simulink model "crf_ut"  (Simulink 8.1)
settings: Solver=FixedStepDiscrete  StartTime=0.0  StopTime=10  FixedStep=0.005  RelTol=1e-3
PostLoadFcn:
  | , if any(exist('dsrtsu_mdlpostloadfcn', 'file') == [2, 3, 6]), try dsrtsu_mdlpostloadfcn('Execute', bdroot); catch fprintf('Error in PostLoadFcn (dsrtsu_mdlpostloadfcn) for model "%s":\n %s\n', bdroot, lasterr); end, end,
libraries: siltestlib x9, crf x1
settings Model: DSRTSU_INTERNAL_RTI_VER=450  DSRTSU_INTERNAL_RTI_TYPE=rti1401  RTICANMMDATA=struct('GeneralSetupData',struct('modelroot','D:\ELN150201_TAIWAN\trunk\AdasDragon\software\sw_development\arch\app\jud','generalsettings',struct('filesettings',struct('destfolder',struct('Name','RTICANMM_FILES','Check',1),'buildfolder',struct('Name','.','Check',1),'AbsDestfolder',struct('Name','D:\ELN150201_TAIWAN\trunk\AdasDragon\software\sw_development\arch\app\jud\RTICANMM_FILES'),'AbsBuildfolder',struct('Name','D:\ELN150201_TAIWAN\trunk\AdasDragon\software\sw_development\arch\app\jud'))),'options',struct('addpaths',1,'rmpaths',1,'addtrcexclusion',logical(1),'cannavigator',struct('checkmonitoring',0),'show_usrtrc',0,'use_usrtrc',0),'advanced',struct('options',[1 1 1 1 1 1 1 1 1 1 1 1 1 1 1 1 1 1 1 1 1 1 1 1 1 1 1 1 1 1 1 1 1 1 1 1 1 1 1 1 1 1 1 1 1 1 1 1 1 1 1 1 1 1 1 1 1 1 1 1 1 1 1 1 1 1 1 1 1 1 1 1 1 1 1 1 1 1 1 1 1 1 1 1 1 1 1 1 1 1 1 1 1 1 1 1 1 1 1 1]),'MPSetup',{{}},'modelname','crf_ut','block','crf_ut'))  DSRTSU_INTERNAL_RTIFPGA=40  Creator=AT015411  LastModifiedBy=AT015555  BufferReuse=off
settings DataIOCC: SignalLoggingSaveFormat=Dataset
settings OptimizationCC: BlockReduction=off  OptimizeBlockIOStorage=off  BufferReuse=off  ExpressionFolding=off  ExpressionDepthLimit=128  LocalBlockOutputs=off
settings DebuggingCC: FcnCallInpInsideContextMsg=EnableAllAsError
settings HardwareCC: ProdIntDivRoundTo=Zero  ProdEndianess=BigEndian  ProdHWDeviceType=Generic->Custom  TargetIntDivRoundTo=Zero  TargetEndianess=BigEndian  TargetHWDeviceType=Generic->Custom
settings RTWCC: SystemTargetFile=rti1005.tlc  MakeCommand=make_rti  TemplateMakefile=rti1005.tmf  Description=dSPACE DS1005 Hardware Platform  ProcessScript=rti1005_make_rtw_hook
settings STFCustomTargetCC: CodeReplacementLibrary=ANSI_C  ParMdlRefBuildCompliant=on  GeneratePreprocessorConditionals=Disable all  MatFileLogging=on  SystemTargetFile=rti1005.tlc
settings GRTTargetCC: CompOptLevelCompliant=off  ConcurrentExecutionCompliant=off  ExtModeMexFile=noextcomm
settings CustomProperty: DataType=RTWOptions_EnumType_C__Program Files (x86)_dSPACE RCPHIL 2014-B_MATLAB_RTI_RTI1401_TLC_rti1005_1InitialSimState  Value=RUN
settings EnumStrPairs: String=RUN

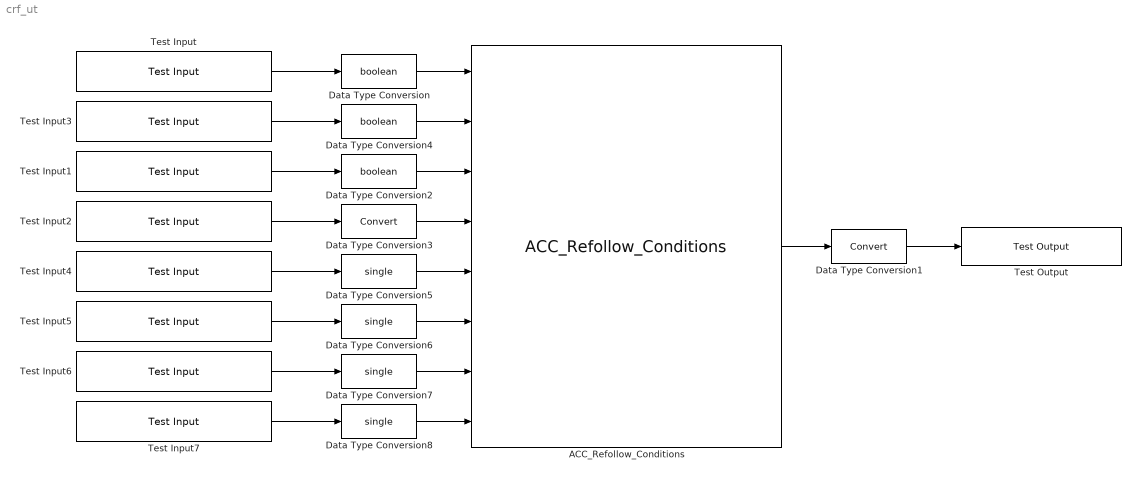
== system crf_ut ==
  ACC_Refollow_Conditions : crf/ACC_Refollow_Conditions
  Data Type Conversion : DataTypeConversion  OutDataTypeStr=boolean
  Data Type Conversion1 : DataTypeConversion
  Data Type Conversion2 : DataTypeConversion  OutDataTypeStr=boolean
  Data Type Conversion3 : DataTypeConversion
  Data Type Conversion4 : DataTypeConversion  OutDataTypeStr=boolean
  Data Type Conversion{5..8} (4 alike) : DataTypeConversion  OutDataTypeStr=single
  Test Input : siltestlib/Test Input  varname=VJUD_ACCVehReadyToStart_flg  sampletime=0.005
  Test Input1 : siltestlib/Test Input  varname=VDINR_DriverBrakPedalOn_flg  sampletime=0.005
  Test Input2 : siltestlib/Test Input  varname=VDINR_ParkBrakeBindSta_enum  sampletime=0.005
  Test Input3 : siltestlib/Test Input  varname=VIFO_ACCTargetVehAssigned_flg  sampletime=0.005
  Test Input4 : siltestlib/Test Input  varname=VIFO_ACCTargetVehRelSpeedX_mps  sampletime=0.005
  Test Input5 : siltestlib/Test Input  varname=VIFO_ACCVehClearance_m  sampletime=0.005
  Test Input6 : siltestlib/Test Input  varname=VACC_DesiredDistancePrev_m  sampletime=0.005
  Test Input7 : siltestlib/Test Input  varname=VACC_StandstillClearancePrev_m  sampletime=0.005
  Test Output : siltestlib/Test Output  varname=VJUD_ACCRefollowReq_flg  sampletime=-1
  wires:
  Data Type Conversion1/1 -> Test Output/1
  Test Input/1 -> Data Type Conversion/1
  Test Input1/1 -> Data Type Conversion2/1
  Data Type Conversion/1 -> ACC_Refollow_Conditions/1
  Data Type Conversion4/1 -> ACC_Refollow_Conditions/2
  ACC_Refollow_Conditions/1 -> Data Type Conversion1/1
  Test Input2/1 -> Data Type Conversion3/1
  Data Type Conversion2/1 -> ACC_Refollow_Conditions/3
  Data Type Conversion3/1 -> ACC_Refollow_Conditions/4
  Test Input3/1 -> Data Type Conversion4/1
  Test Input4/1 -> Data Type Conversion5/1
  Data Type Conversion5/1 -> ACC_Refollow_Conditions/5
  Test Input5/1 -> Data Type Conversion6/1
  Data Type Conversion6/1 -> ACC_Refollow_Conditions/6
  Test Input6/1 -> Data Type Conversion7/1
  Data Type Conversion7/1 -> ACC_Refollow_Conditions/7
  Test Input7/1 -> Data Type Conversion8/1
  Data Type Conversion8/1 -> ACC_Refollow_Conditions/8
